simulink model "mpc_pathFollowingMod"  (R2024a)
settings: Solver=VariableStepAuto  StartTime=0.0  StopTime=10.0  RelTol=1e-3
PreLoadFcn:
  | load('pathFollowingUtil\pfcsubsystem_data.mat');
  | load('pathFollowingUtil\mpc_base.mat');
values from neighbouring files (symbols this model uses):
  Cf = evalin('base','Cf')    [helperSLTrajectoryFollowerWithRRScenarioSetup.m]
  Cr = evalin('base','Cr')    [helperSLTrajectoryFollowerWithRRScenarioSetup.m]
  Iz = evalin('base','Iz')    [helperSLTrajectoryFollowerWithRRScenarioSetup.m]
  lf = evalin('base','lf')    [helperSLTrajectoryFollowerWithRRScenarioSetup.m]
  lr = evalin('base','lr')    [helperSLTrajectoryFollowerWithRRScenarioSetup.m]
  m = worldActors(idx).actor_runtime.pose.matrix    [helperSLTrajectoryFollowerWithRRScenarioSetup.m]
  numReferencePose = 1    [HelperReferencePoseOnPath.m]
  pfcsubsystem_data =     [pfcsubsystem_data.mat]
undefined symbols (not defined in the file or in its folder): control_timeStep, DefaultSpacing, E_mpc, F_mpc, hasLag, InitialLongVel, NumEgoStates, sizeExNumSS, tau, tau2
libraries: mpcsigdimcheck_private x19, mpclib x3, simulink x2, sharedTrackingLibrary x1
(part 2 of 2)

== matlab function mpc_pathFollowingMod/PFC subsystem/update plant model ==
  data: Vx input; u input; A output; x input; Ts input; B output; C output; D output; U output; Y output; X output; DX output; m parameter; Iz parameter; lf parameter; lr parameter; Cf parameter; Cr parameter; tau parameter; tau2 parameter; sizeExNumSS parameter
function [A,B,C,D,U,Y,X,DX] = fcn(Vx,u,x,Ts,m, Iz, lf, lr, Cf, Cr, tau, tau2, sizeExNumSS)
% % Sample time
psi_dot = x(5+sizeExNumSS);
lag = tau2;
% if tau2 > eps
%     if numel(x) >= 6
%         psi_dot = x(6);
%     end
%     lag = tau2;
% else
%     if numel(x) >= 5
%         psi_dot = x(5);
%     end
% end
% Continuous-time model
Ac = [0 1 psi_dot 0 0 0;
     0 -1/tau 0 0 0 0;
     0 0 -(2*Cf+2*Cr)/(m*Vx) 0 -Vx-(2*Cf*lf - 2*Cr*lr)/(m*Vx) 0;
     0 0 0 0 1 0;
     0 0 -(2*Cf*lf-2*Cr*lr)/(Iz*Vx) 0 -(2*Cf*lf^2+2*Cr*lr^2)/(Iz*Vx) 0;
     0 0 1 Vx 0 0];
Bc = [0 0; 1/tau 0; 0 2*Cf/m; 0 0; 0 2*Cf*lf/Iz; 0 0];
% Cc = [1 0 0 0 0 0; 0 0 0 0 0 1; 0 0 0 1 0 0];
Cc = [1 0 0 0 0 0; 0 0 0 0 0 1; 0 0 0 1 0 0; 0 0 0 0 1 0];
Dc = zeros(size(Cc,1),size(Bc,2));

% As = zeros(6+sizeExNumSS, 6+sizeExNumSS);
% Bs = zeros(6+sizeExNumSS, 2);
% Cs = zeros(4, 6+sizeExNumSS);
% Ds = zeros(4, 2);
if  sizeExNumSS == 1
    Atemp = Ac; Btemp = Bc; Ctemp = Cc; Dtemp = Dc;
    Al = -1/lag; Bl = [0, 1/lag]; Cl = [0; 1]; Dl = [1, 0; 0, 0];
    As = [Al, zeros(1, size(Atemp, 2)); Btemp*Cl, Atemp];
    Bs = [Bl; Btemp*Dl];
    Cs = [Dtemp * Cl, Ctemp];
    Ds = Dtemp * Dl;
else
    As = Ac; Bs = Bc; Cs = Cc; Ds = Dc;
end

% Discretize the continuous-time model using zero-order hold 
% % on the inputs and a sample time of Ts seconds
% nx = size(As,1);
% nu = size(Bs,2);
nx = 6+sizeExNumSS;
nu = size(Bs,2);
M = expm([[As Bs]*Ts; zeros(nu,nx+nu)]);
A = M(1:nx,1:nx);
B = M(1:nx,nx+1:nx+nu);
C = Cs;
D = Ds;

% Nominal conditions for discrete-time plant
X = x;
U = u;
Y = C*x + D*u;
DX = A*x+B*u-x;

% X = zeros(nx, 1);
% U = zeros(nu, 1);
% Y = zeros(Cc, 2);

== matlab function mpc_pathFollowingMod/PFC subsystem/Data Processing for MPC Controller/DataTypeConversion_extmv ==
  data: u input size=[2 1]; y output; isDouble parameter
function y = fcn(u,isDouble)
if isDouble
    if isa(u,'double')
        y = u;
    else
        y = double(u);
    end
else
    if isa(u,'single')
        y = u;
    else
        y = single(u);
    end
end

== matlab function mpc_pathFollowingMod/ref2err_MATLABFunction ==
  data: refPose input size=[numReferencePose, 3]; refY output; currPose input; refTheta output
function [refY, refTheta] = fcn(refPose, currPose)
% lateral deviation
% Ego vehicle lateral deviation in meters from the centerline of the lane.
% The lateral deviation e1 is positive when the ego vehicle is to the right of the centerline and negative when the ego vehicle is to the left of the centerline.
% yaw_diff
% Ego vehicle longitudinal axis angle in radians from the centerline of the lane, defined as:
% Here, θe is the ego vehicle angle and θc is the centerline angle, with both angles defined in the global coordinate frame.
yaw = deg2rad(currPose(3));
rotm = [cos(yaw ), -sin(yaw ); sin(yaw ) cos(yaw )];
rotm_inv = transpose(rotm);

% refXY = transpose(rotm_inv * transpose(refPose(:, 1:2)));
refXY = transpose(rotm_inv * transpose(refPose(:, 1:2) - currPose(1:2)'));
refY = refXY(:, 2);
refTheta = deg2rad(refPose(:,3) - currPose(3));

% refY = refPose(:,2);
% refTheta = deg2rad(refPose(:,3));
